simulink model "DAL_Sat_HW_v5"  (R2021b)
settings: Solver=FixedStepAuto  StartTime=0.0  StopTime=Inf  RelTol=1e-3  EnableMultiTasking=on
undefined symbols (not defined in the file): magnitude
libraries: arduinolib x11
settings Model: ExtModeTrigDuration=2  Creator=diego  LastModifiedBy=diego
settings OptimizationCC: EnhancedBackFolding=on  PassReuseOutputArgsAs=Individual arguments  ZeroExternalMemoryAtStartup=off  ZeroInternalMemoryAtStartup=off  MaxStackSize=64  OptimizeBlockOrder=speed  DifferentSizesBufferReuse=on  EfficientTunableParamExpr=on
settings DebuggingCC: ParameterTunabilityLossMsg=error
settings HardwareCC: ProdBitPerInt=16  ProdBitPerPointer=16  ProdBitPerSizeT=16  ProdBitPerPtrDiffT=16  ProdLargestAtomicFloat=None  ProdWordSize=8  ProdHWDeviceType=Atmel->AVR
settings SFSimCC: MATLABDynamicMemAlloc=off
settings RTWCC: Description=Embedded Coder  SystemTargetFile=ert.tlc  HardwareBoard=Arduino Uno  TemplateMakefile=ert_default_tmf  Toolchain=Arduino AVR  BuildConfiguration=Faster Runs
settings CodeAppCC: ForceParamTrailComments=on  IgnoreCustomStorageClasses=off  OperatorAnnotations=on  SimulinkDataObjDesc=on  SFDataObjDesc=on  InsertBlockDesc=on
settings ERTTargetCC: SupportContinuousTime=on  SupportVariableSizeSignals=on  ExtModeTransport=3  ExtModeStaticAlloc=on  ExtModeStaticAllocSize=250  ExtModeMexFile=ext_xcp  ExtModeIntrfLevel=Level2 - Open

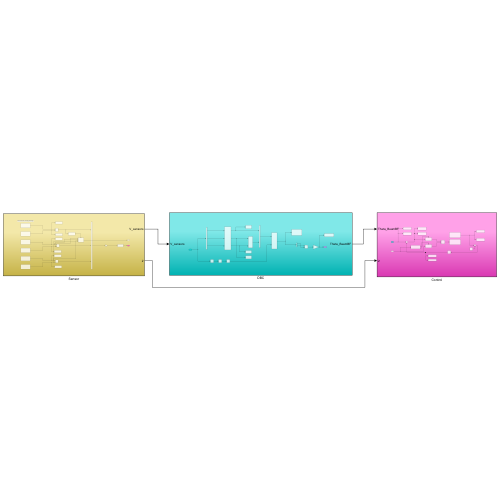
[thumbnail: Simulink's stored preview of the top-level diagram]
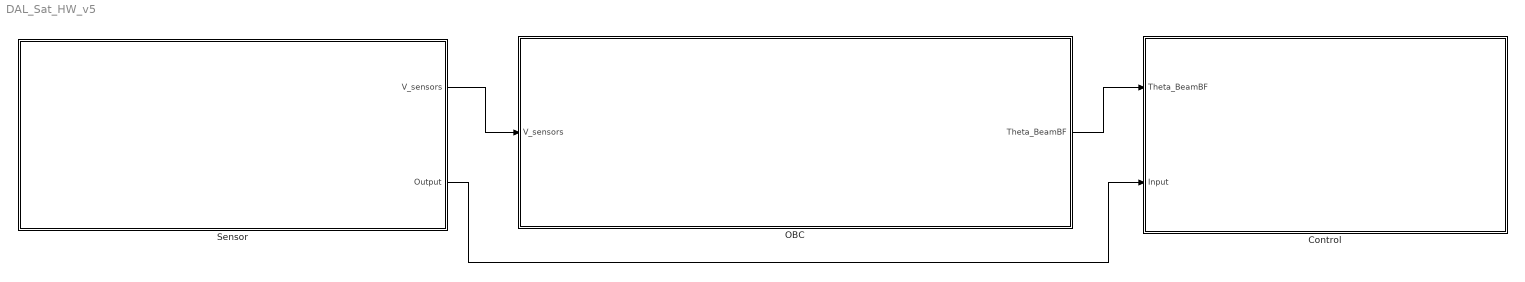
== system DAL_Sat_HW_v5 ==
  Control : Subsystem
  OBC : Subsystem
  Sensor : Subsystem
  wires:
  OBC/1(Theta_BeamBF) -> Control/1(Theta_BeamBF)
  Sensor/1(V_sensors) -> OBC/1(V_sensors)
  Sensor/2(Output) -> Control/2(Input)

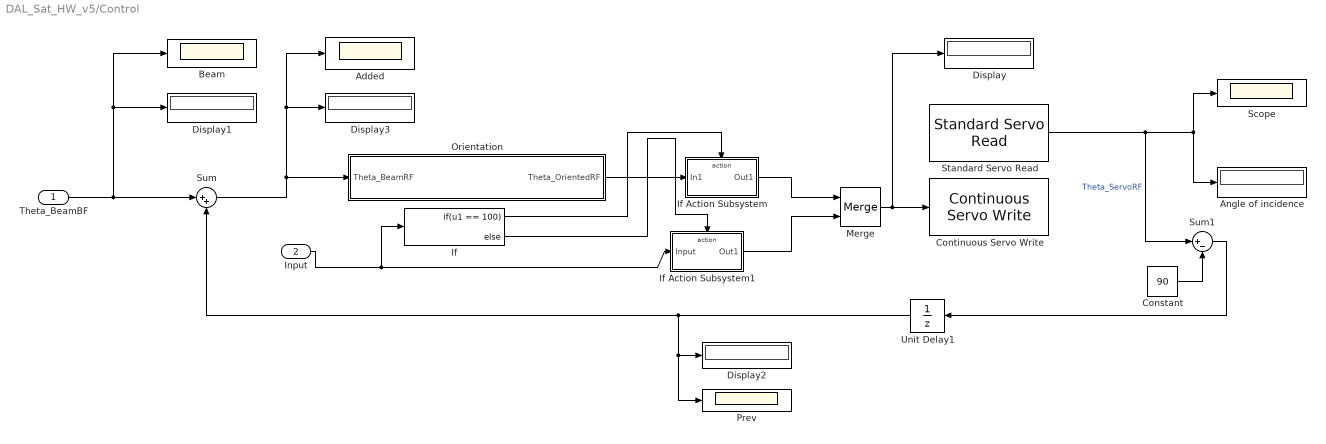
== system DAL_Sat_HW_v5/Control ==
  Theta_BeamBF : Inport
  Input : Inport  Port=2
  Added : Scope
  Angle of incidence : Display
  Beam : Scope
  Constant : Constant  Value=90
  Continuous Servo Write : arduinolib/Continuous Servo Write  pinNumber=9  ServoIndex=0  blockPlatform=ARDUINO
      settings: SourceProductBaseCode=ARDUINO
  Display{,1..3} (4 alike) : Display
  If : If  IfExpression=u1 == 100
  If Action Subsystem : Subsystem  TreatAsAtomicUnit=on
  If Action Subsystem1 : Subsystem  TreatAsAtomicUnit=on
  Merge : Merge
  Orientation : Subsystem
  Prev : Scope
  Scope : Scope
  Standard Servo Read : arduinolib/Standard Servo Read  pinNumber=9  SampleTime=0.1  ServoIndex=0  blockPlatform=ARDUINO
      settings: SourceProductBaseCode=ARDUINO
  Sum : Sum  Inputs=|++
  Sum1 : Sum  Inputs=|+-
  Unit Delay1 : UnitDelay  SampleTime=-1  HasFrameUpgradeWarning=on
  wires:
  Standard Servo Read/1 -> Scope/1, Angle of incidence/1, Sum1/1  "Theta_ServoRF"
  Unit Delay1/1 -> Prev/1, Display2/1, Sum/2
  Theta_BeamBF/1 -> Beam/1, Display1/1, Sum/1
  Sum1/1 -> Unit Delay1/1
  Constant/1 -> Sum1/2
  Sum/1 -> Display3/1, Added/1, Orientation/1(Theta_BeamRF)
  Merge/1 -> Display/1, Continuous Servo Write/1
  Input/1 -> If/1, If Action Subsystem1/1(Input)
  If/1 -> If Action Subsystem/Action
  If/2 -> If Action Subsystem1/Action
  If Action Subsystem/1(Out1) -> Merge/1
  If Action Subsystem1/1(Out1) -> Merge/2
  Orientation/1(Theta_OrientedRF) -> If Action Subsystem/1(In1)

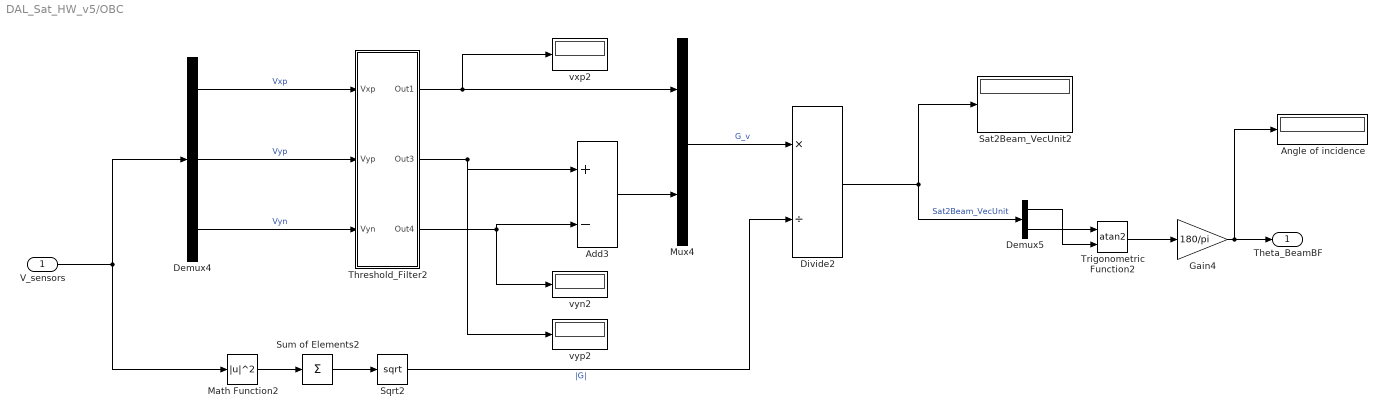
== system DAL_Sat_HW_v5/OBC ==
  V_sensors : Inport
  Add3 : Sum  Inputs=+|-
  Angle of incidence : Display
  Demux4 : Demux  Outputs=3
  Demux5 : Demux  Outputs=2
  Divide2 : Product  Inputs=*/
  Gain4 : Gain  Gain=180/pi
  Math Function2 : Math  Operator=magnitude^2  OutputSignalType=real  SaturateOnIntegerOverflow=on
  Mux4 : Mux  Inputs=2
  Sat2Beam_VecUnit2 : Display
  Sqrt2 : Sqrt  SaturateOnIntegerOverflow=on
  Sum of Elements2 : Sum  Inputs=+
  Threshold_Filter2 : Subsystem
  Trigonometric Function2 : Trigonometry  Operator=atan2
  vxp2 : Display
  vyn2 : Display
  vyp2 : Display
  Theta_BeamBF : Outport
  wires:
  V_sensors/1 -> Demux4/1, Math Function2/1
  Demux4/2 -> Threshold_Filter2/2(Vyp)  "Vyp"
  Trigonometric Function2/1 -> Gain4/1
  Threshold_Filter2/1(Out1) -> vxp2/1, Mux4/1
  Divide2/1 -> Sat2Beam_VecUnit2/1, Demux5/1  "Sat2Beam_VecUnit"
  Demux4/3 -> Threshold_Filter2/3(Vyn)  "Vyn"
  Sqrt2/1 -> Divide2/2  "|G|"
  Demux5/1 -> Trigonometric Function2/2
  Demux4/1 -> Threshold_Filter2/1(Vxp)  "Vxp"
  Threshold_Filter2/3(Out4) -> vyn2/1, Add3/2
  Add3/1 -> Mux4/2
  Threshold_Filter2/2(Out3) -> vyp2/1, Add3/1
  Mux4/1 -> Divide2/1  "G_v"
  Demux5/2 -> Trigonometric Function2/1
  Sum of Elements2/1 -> Sqrt2/1
  Math Function2/1 -> Sum of Elements2/1
  Gain4/1 -> Angle of incidence/1, Theta_BeamBF/1

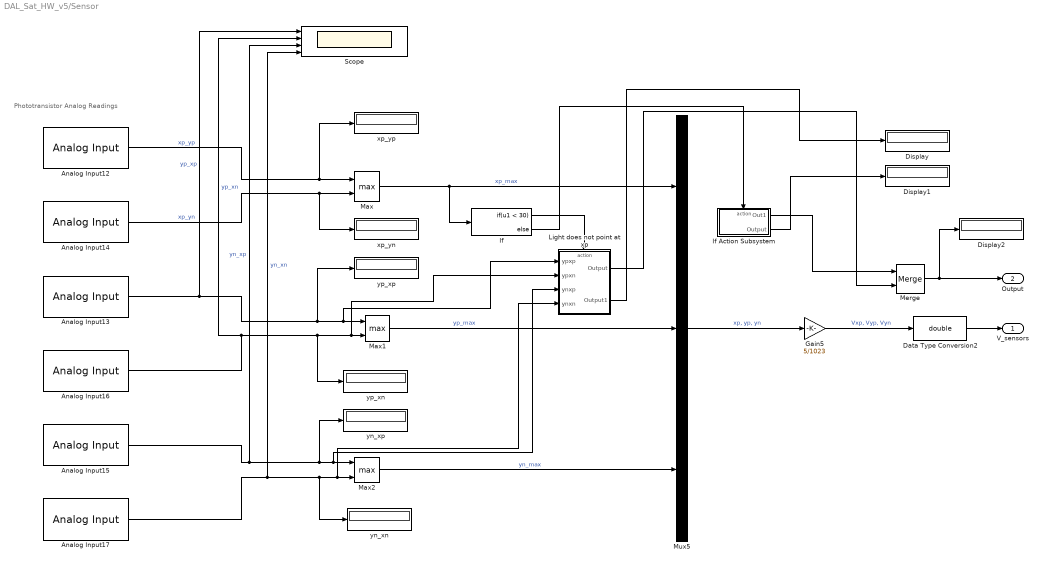
== system DAL_Sat_HW_v5/Sensor ==
  note: Phototransistor Analog Readings
  Analog Input12 : arduinolib/Analog Input  pinNumber=2  ReadResultsOnly=off  ConversionTriggerSource=Software  ExternalTriggerType=uint32( 0 )  OutputDataType=uint16  EnableConversionCompleteNotify=off  EnableOuputStatus=off  SampleTime=-1  blockPlatform=arduino
  Analog Input13 : arduinolib/Analog Input  pinNumber=1  ReadResultsOnly=off  ConversionTriggerSource=Software  ExternalTriggerType=uint32( 0 )  OutputDataType=uint16  EnableConversionCompleteNotify=off  EnableOuputStatus=off  SampleTime=-1  blockPlatform=arduino
  Analog Input14 : arduinolib/Analog Input  pinNumber=3  ReadResultsOnly=off  ConversionTriggerSource=Software  ExternalTriggerType=uint32( 0 )  OutputDataType=uint16  EnableConversionCompleteNotify=off  EnableOuputStatus=off  SampleTime=-1  blockPlatform=arduino
  Analog Input15 : arduinolib/Analog Input  pinNumber=4  ReadResultsOnly=off  ConversionTriggerSource=Software  ExternalTriggerType=uint32( 0 )  OutputDataType=uint16  EnableConversionCompleteNotify=off  EnableOuputStatus=off  SampleTime=-1  blockPlatform=arduino
  Analog Input16 : arduinolib/Analog Input  pinNumber=0  ReadResultsOnly=off  ConversionTriggerSource=Software  ExternalTriggerType=uint32( 0 )  OutputDataType=uint16  EnableConversionCompleteNotify=off  EnableOuputStatus=off  SampleTime=-1  blockPlatform=arduino
  Analog Input17 : arduinolib/Analog Input  pinNumber=5  ReadResultsOnly=off  ConversionTriggerSource=Software  ExternalTriggerType=uint32( 0 )  OutputDataType=uint16  EnableConversionCompleteNotify=off  EnableOuputStatus=off  SampleTime=-1  blockPlatform=arduino
  Data Type Conversion2 : DataTypeConversion  OutDataTypeStr=double
  Display : Display
  Display1 : Display
  Display2 : Display
  Gain5 : Gain  Gain=5/1023
  If : If  IfExpression=u1 < 30
  If Action Subsystem : Subsystem  TreatAsAtomicUnit=on
  Light does not point at xp : Subsystem  TreatAsAtomicUnit=on
  Max : MinMax  Function=max  Inputs=2
  Max1 : MinMax  Function=max  Inputs=2
  Max2 : MinMax  Function=max  Inputs=2
  Merge : Merge
  Mux5 : Mux  Inputs=3
  Scope : Scope  NumInputPorts=4
  xp_yn : Display
  xp_yp : Display
  yn_xn : Display
  yn_xp : Display
  yp_xn : Display
  yp_xp : Display
  V_sensors : Outport
  Output : Outport  Port=2
  wires:
  Analog Input12/1 -> Max/1, xp_yp/1  "xp_yp"
  Analog Input14/1 -> Max/2, xp_yn/1  "xp_yn"
  Analog Input13/1 -> Light does not point at xp/1(ypxp), Max1/1, yp_xp/1, Scope/1  "yp_xp"
  Max2/1 -> Mux5/3  "yn_max"
  Max/1 -> If/1, Mux5/1  "xp_max"
  Analog Input15/1 -> Light does not point at xp/3(ynxp), Max2/1, yn_xp/1, Scope/3  "yn_xp"
  Analog Input16/1 -> Light does not point at xp/2(ypxn), Max1/2, yp_xn/1, Scope/2  "yp_xn"
  Analog Input17/1 -> Light does not point at xp/4(ynxn), Max2/2, yn_xn/1, Scope/4  "yn_xn"
  Max1/1 -> Mux5/2  "yp_max"
  Mux5/1 -> Gain5/1  "xp, yp, yn"
  Gain5/1 -> Data Type Conversion2/1  "Vxp, Vyp, Vyn"
  Data Type Conversion2/1 -> V_sensors/1
  If/1 -> Light does not point at xp/Action
  Merge/1 -> Display2/1, Output/1
  If Action Subsystem/1(Out1) -> Merge/1
  Light does not point at xp/1(Output) -> Merge/2
  If/2 -> If Action Subsystem/Action
  Light does not point at xp/2(Output1) -> Display/1
  If Action Subsystem/2(Output) -> Display1/1

== system DAL_Sat_HW_v5/Control/If Action Subsystem ==
  In1 : Inport
  Action Port : ActionPort  ActionPortLabel=if(u1 == 100)
  Out1 : Outport
  wires:
  In1/1 -> Out1/1

== system DAL_Sat_HW_v5/Control/If Action Subsystem1 ==
  Input : Inport
  Action Port : ActionPort  ActionPortLabel=else
  Out1 : Outport
  wires:
  Input/1 -> Out1/1

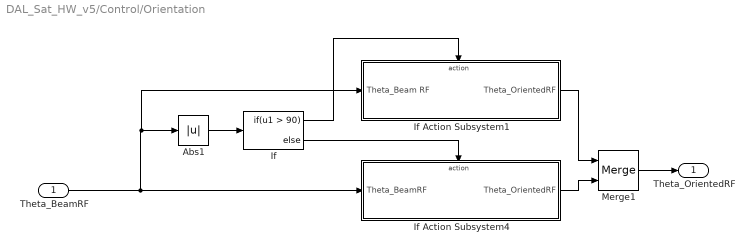
== system DAL_Sat_HW_v5/Control/Orientation ==
  Theta_BeamRF : Inport
  Abs1 : Abs
  If : If  IfExpression=u1 > 90
  If Action Subsystem1 : Subsystem  TreatAsAtomicUnit=on
  If Action Subsystem4 : Subsystem  TreatAsAtomicUnit=on
  Merge1 : Merge
  Theta_OrientedRF : Outport
  wires:
  If Action Subsystem1/1(Theta_OrientedRF) -> Merge1/1
  Merge1/1 -> Theta_OrientedRF/1
  If/2 -> If Action Subsystem4/Action
  If/1 -> If Action Subsystem1/Action
  Abs1/1 -> If/1
  Theta_BeamRF/1 -> If Action Subsystem1/1(Theta_Beam	RF), Abs1/1, If Action Subsystem4/1(Theta_BeamRF)
  If Action Subsystem4/1(Theta_OrientedRF) -> Merge1/2

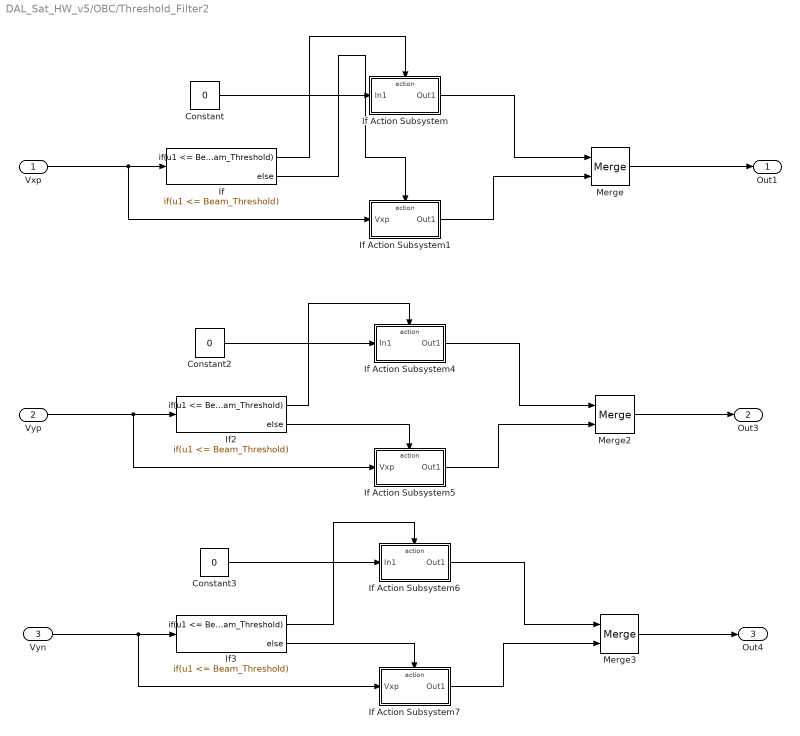
== system DAL_Sat_HW_v5/OBC/Threshold_Filter2 ==
  Vxp : Inport
  Vyp : Inport  Port=2
  Vyn : Inport  Port=3
  Constant : Constant  Value=0
  Constant2 : Constant  Value=0
  Constant3 : Constant  Value=0
  If : If  IfExpression=u1 <= Beam_Threshold
  If Action Subsystem : Subsystem  TreatAsAtomicUnit=on
  If Action Subsystem1 : Subsystem  TreatAsAtomicUnit=on
  If Action Subsystem4 : Subsystem  TreatAsAtomicUnit=on
  If Action Subsystem5 : Subsystem  TreatAsAtomicUnit=on
  If Action Subsystem6 : Subsystem  TreatAsAtomicUnit=on
  If Action Subsystem7 : Subsystem  TreatAsAtomicUnit=on
  If2 : If  IfExpression=u1 <= Beam_Threshold
  If3 : If  IfExpression=u1 <= Beam_Threshold
  Merge : Merge
  Merge2 : Merge
  Merge3 : Merge
  Out1 : Outport
  Out3 : Outport  Port=2
  Out4 : Outport  Port=3
  wires:
  Vxp/1 -> If Action Subsystem1/1(Vxp), If/1
  If/1 -> If Action Subsystem/Action
  If Action Subsystem/1(Out1) -> Merge/1
  If/2 -> If Action Subsystem1/Action
  If Action Subsystem1/1(Out1) -> Merge/2
  Merge/1 -> Out1/1
  Constant/1 -> If Action Subsystem/1(In1)
  Vyp/1 -> If2/1, If Action Subsystem5/1(Vxp)
  If2/2 -> If Action Subsystem5/Action
  If2/1 -> If Action Subsystem4/Action
  If Action Subsystem4/1(Out1) -> Merge2/1
  If Action Subsystem5/1(Out1) -> Merge2/2
  Constant2/1 -> If Action Subsystem4/1(In1)
  Merge2/1 -> Out3/1
  Vyn/1 -> If3/1, If Action Subsystem7/1(Vxp)
  Merge3/1 -> Out4/1
  If Action Subsystem7/1(Out1) -> Merge3/2
  If3/2 -> If Action Subsystem7/Action
  If Action Subsystem6/1(Out1) -> Merge3/1
  Constant3/1 -> If Action Subsystem6/1(In1)
  If3/1 -> If Action Subsystem6/Action

== system DAL_Sat_HW_v5/Sensor/If Action Subsystem ==
  Action Port : ActionPort  ActionPortLabel=else
  Constant : Constant  Value=100
  Out1 : Outport
  Output : Outport  Port=2
  wires:
  Constant/1 -> Output/1, Out1/1

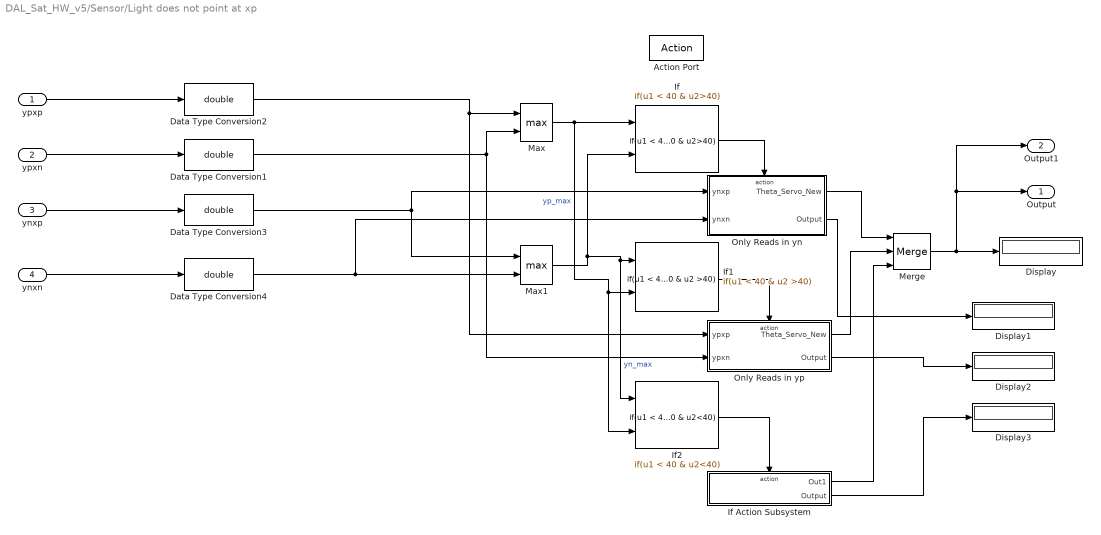
== system DAL_Sat_HW_v5/Sensor/Light does not point at xp ==
  ypxp : Inport
  ypxn : Inport  Port=2
  ynxp : Inport  Port=3
  ynxn : Inport  Port=4
  Action Port : ActionPort  ActionPortLabel=if(u1 < 30)
  Data Type Conversion{1..4} (4 alike) : DataTypeConversion  OutDataTypeStr=double
  Display{,1..3} (4 alike) : Display
  If : If  NumInputs=2  IfExpression=u1 < 40 & u2>40  ShowElse=off
  If Action Subsystem : Subsystem  TreatAsAtomicUnit=on
  If1 : If  NumInputs=2  IfExpression=u1 < 40 & u2 >40  ShowElse=off
  If2 : If  NumInputs=2  IfExpression=u1 < 40 & u2<40  ShowElse=off
  Max : MinMax  Function=max  Inputs=2
  Max1 : MinMax  Function=max  Inputs=2
  Merge : Merge  Inputs=3
  Only Reads in yn : Subsystem  TreatAsAtomicUnit=on
  Only Reads in yp : Subsystem  TreatAsAtomicUnit=on
  Output : Outport
  Output1 : Outport  Port=2
  wires:
  Max/1 -> If2/2, If1/2, If/1  "yp_max"
  Max1/1 -> If/2, If2/1, If1/1  "yn_max"
  Only Reads in yn/1(Theta_Servo_New) -> Merge/1
  Only Reads in yp/1(Theta_Servo_New) -> Merge/2
  Merge/1 -> Output1/1, Output/1, Display/1
  If/1 -> Only Reads in yn/Action
  If1/1 -> Only Reads in yp/Action
  If2/1 -> If Action Subsystem/Action
  If Action Subsystem/1(Out1) -> Merge/3
  Only Reads in yn/2(Output) -> Display1/1
  Only Reads in yp/2(Output) -> Display2/1
  If Action Subsystem/2(Output) -> Display3/1
  Data Type Conversion2/1 -> Only Reads in yp/1(ypxp), Max/1
  Data Type Conversion1/1 -> Only Reads in yp/2(ypxn), Max/2
  Data Type Conversion3/1 -> Max1/1, Only Reads in yn/1(ynxp)
  ypxn/1 -> Data Type Conversion1/1
  ypxp/1 -> Data Type Conversion2/1
  ynxn/1 -> Data Type Conversion4/1
  ynxp/1 -> Data Type Conversion3/1
  Data Type Conversion4/1 -> Only Reads in yn/2(ynxn), Max1/2

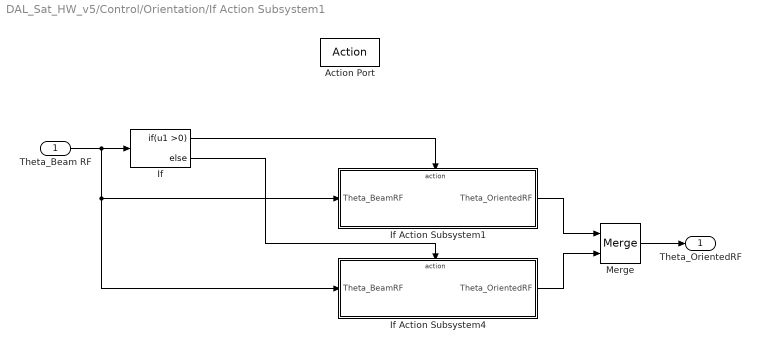
== system DAL_Sat_HW_v5/Control/Orientation/If Action Subsystem1 ==
  Theta_Beam	RF : Inport
  Action Port : ActionPort  ActionPortLabel=if(u1 > 90)
  If : If  IfExpression=u1 >0
  If Action Subsystem1 : Subsystem  TreatAsAtomicUnit=on
  If Action Subsystem4 : Subsystem  TreatAsAtomicUnit=on
  Merge : Merge
  Theta_OrientedRF : Outport
  wires:
  Theta_Beam	RF/1 -> If Action Subsystem4/1(Theta_BeamRF), If Action Subsystem1/1(Theta_BeamRF), If/1
  If/1 -> If Action Subsystem1/Action
  If/2 -> If Action Subsystem4/Action
  If Action Subsystem1/1(Theta_OrientedRF) -> Merge/1
  If Action Subsystem4/1(Theta_OrientedRF) -> Merge/2
  Merge/1 -> Theta_OrientedRF/1

== system DAL_Sat_HW_v5/Control/Orientation/If Action Subsystem4 ==
  Theta_BeamRF : Inport
  Action Port : ActionPort  ActionPortLabel=else
  Theta_OrientedRF : Outport
  wires:
  Theta_BeamRF/1 -> Theta_OrientedRF/1

== system DAL_Sat_HW_v5/OBC/Threshold_Filter2/If Action Subsystem ==
  In1 : Inport
  Action Port : ActionPort  ActionPortLabel=if(u1 <= Beam_Threshold)
  Out1 : Outport
  wires:
  In1/1 -> Out1/1

== system DAL_Sat_HW_v5/OBC/Threshold_Filter2/If Action Subsystem1 ==
  Vxp : Inport
  Action Port : ActionPort  ActionPortLabel=else
  Out1 : Outport
  wires:
  Vxp/1 -> Out1/1

== system DAL_Sat_HW_v5/OBC/Threshold_Filter2/If Action Subsystem4 ==
  In1 : Inport
  Action Port : ActionPort  ActionPortLabel=if(u1 <= Beam_Threshold)
  Out1 : Outport
  wires:
  In1/1 -> Out1/1

== system DAL_Sat_HW_v5/OBC/Threshold_Filter2/If Action Subsystem5 ==
  Vxp : Inport
  Action Port : ActionPort  ActionPortLabel=else
  Out1 : Outport
  wires:
  Vxp/1 -> Out1/1

== system DAL_Sat_HW_v5/OBC/Threshold_Filter2/If Action Subsystem6 ==
  In1 : Inport
  Action Port : ActionPort  ActionPortLabel=if(u1 <= Beam_Threshold)
  Out1 : Outport
  wires:
  In1/1 -> Out1/1

== system DAL_Sat_HW_v5/OBC/Threshold_Filter2/If Action Subsystem7 ==
  Vxp : Inport
  Action Port : ActionPort  ActionPortLabel=else
  Out1 : Outport
  wires:
  Vxp/1 -> Out1/1

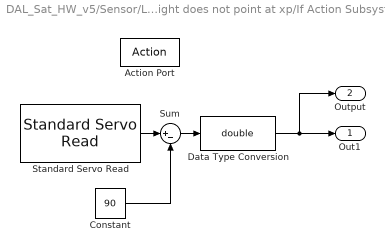
== system DAL_Sat_HW_v5/Sensor/Light does not point at xp/If Action Subsystem ==
  Action Port : ActionPort  ActionPortLabel=if(u1 < 40 & u2<40)
  Constant : Constant  Value=90
  Data Type Conversion : DataTypeConversion  OutDataTypeStr=double
  Standard Servo Read : arduinolib/Standard Servo Read  pinNumber=2  SampleTime=0.1  ServoIndex=1  blockPlatform=ARDUINO
      settings: SourceProductBaseCode=ARDUINO
  Sum : Sum  Inputs=|+-
  Out1 : Outport
  Output : Outport  Port=2
  wires:
  Data Type Conversion/1 -> Output/1, Out1/1
  Standard Servo Read/1 -> Sum/1
  Sum/1 -> Data Type Conversion/1
  Constant/1 -> Sum/2

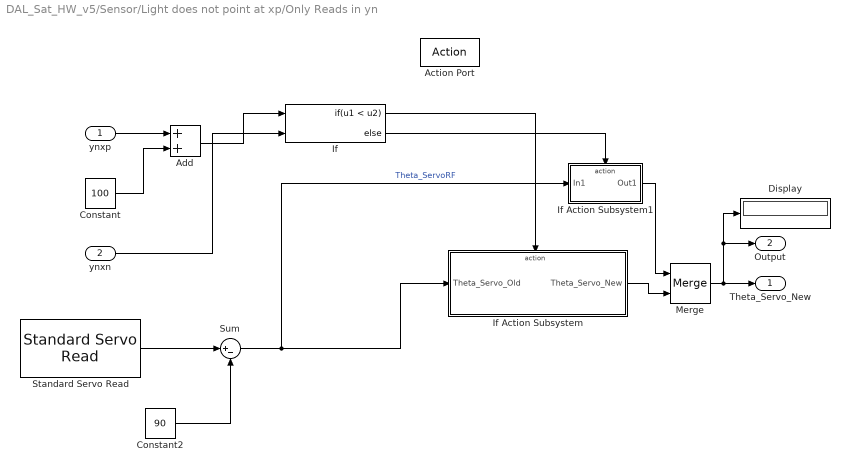
== system DAL_Sat_HW_v5/Sensor/Light does not point at xp/Only Reads in yn ==
  ynxp : Inport
  ynxn : Inport  Port=2
  Action Port : ActionPort  ActionPortLabel=if(u1 < 40 & u2>40)
  Add : Sum
  Constant : Constant  Value=100
  Constant2 : Constant  Value=90
  Display : Display
  If : If  NumInputs=2  IfExpression=u1 < u2
  If Action Subsystem : Subsystem  TreatAsAtomicUnit=on
  If Action Subsystem1 : Subsystem  TreatAsAtomicUnit=on
  Merge : Merge
  Standard Servo Read : arduinolib/Standard Servo Read  pinNumber=9  SampleTime=0.1  ServoIndex=0  blockPlatform=ARDUINO
      settings: SourceProductBaseCode=ARDUINO
  Sum : Sum  Inputs=|+-
  Theta_Servo_New : Outport
  Output : Outport  Port=2
  wires:
  ynxp/1 -> Add/1
  Constant/1 -> Add/2
  Add/1 -> If/1
  ynxn/1 -> If/2
  If/1 -> If Action Subsystem/Action
  If/2 -> If Action Subsystem1/Action
  If Action Subsystem1/1(Out1) -> Merge/1
  If Action Subsystem/1(Theta_Servo_New) -> Merge/2
  Merge/1 -> Display/1, Output/1, Theta_Servo_New/1
  Standard Servo Read/1 -> Sum/1
  Sum/1 -> If Action Subsystem1/1(In1), If Action Subsystem/1(Theta_Servo_Old)  "Theta_ServoRF"
  Constant2/1 -> Sum/2

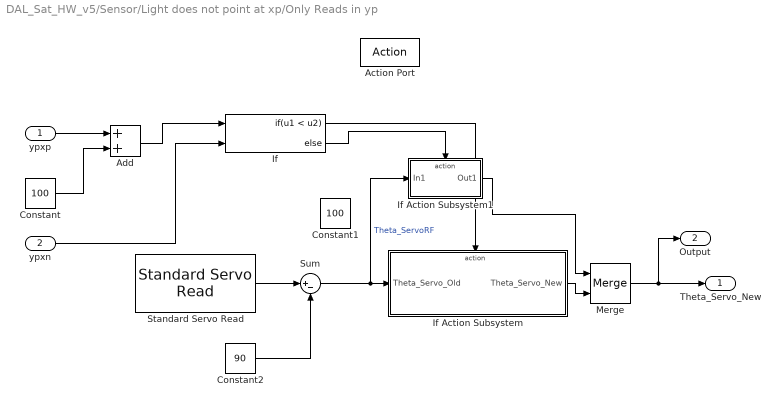
== system DAL_Sat_HW_v5/Sensor/Light does not point at xp/Only Reads in yp ==
  ypxp : Inport
  ypxn : Inport  Port=2
  Action Port : ActionPort  ActionPortLabel=if(u1 < 40 & u2 >40)
  Add : Sum
  Constant : Constant  Value=100
  Constant1 : Constant  Value=100
  Constant2 : Constant  Value=90
  If : If  NumInputs=2  IfExpression=u1 < u2
  If Action Subsystem : Subsystem  TreatAsAtomicUnit=on
  If Action Subsystem1 : Subsystem  TreatAsAtomicUnit=on
  Merge : Merge
  Standard Servo Read : arduinolib/Standard Servo Read  pinNumber=9  SampleTime=0.1  ServoIndex=0  blockPlatform=ARDUINO
      settings: SourceProductBaseCode=ARDUINO
  Sum : Sum  Inputs=|+-
  Theta_Servo_New : Outport
  Output : Outport  Port=2
  wires:
  ypxp/1 -> Add/1
  Constant/1 -> Add/2
  Add/1 -> If/1
  ypxn/1 -> If/2
  If/1 -> If Action Subsystem/Action
  If/2 -> If Action Subsystem1/Action
  Merge/1 -> Output/1, Theta_Servo_New/1
  If Action Subsystem1/1(Out1) -> Merge/1
  If Action Subsystem/1(Theta_Servo_New) -> Merge/2
  Sum/1 -> If Action Subsystem1/1(In1), If Action Subsystem/1(Theta_Servo_Old)  "Theta_ServoRF"
  Standard Servo Read/1 -> Sum/1
  Constant2/1 -> Sum/2

== system DAL_Sat_HW_v5/Control/Orientation/If Action Subsystem1/If Action Subsystem1 ==
  Theta_BeamRF : Inport
  Action Port : ActionPort  ActionPortLabel=if(u1 >0)
  Constant : Constant  Value=180
  Subtract : Sum
  Theta_OrientedRF : Outport
  wires:
  Subtract/1 -> Theta_OrientedRF/1
  Theta_BeamRF/1 -> Subtract/1
  Constant/1 -> Subtract/2

== system DAL_Sat_HW_v5/Control/Orientation/If Action Subsystem1/If Action Subsystem4 ==
  Theta_BeamRF : Inport
  Action Port : ActionPort  ActionPortLabel=else
  Constant : Constant  Value=180
  Subtract : Sum  Inputs=+-
  Theta_OrientedRF : Outport
  wires:
  Theta_BeamRF/1 -> Subtract/1
  Constant/1 -> Subtract/2
  Subtract/1 -> Theta_OrientedRF/1

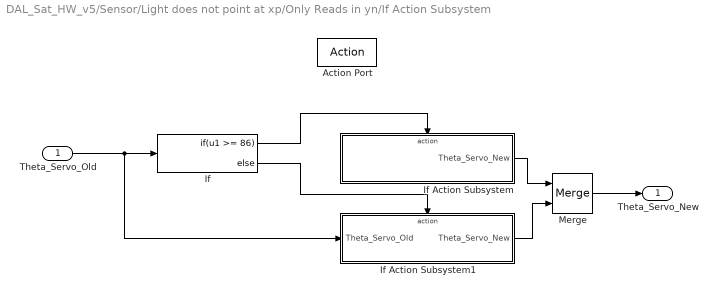
== system DAL_Sat_HW_v5/Sensor/Light does not point at xp/Only Reads in yn/If Action Subsystem ==
  Theta_Servo_Old : Inport
  Action Port : ActionPort  ActionPortLabel=if(u1 < u2)
  If : If  IfExpression=u1 >= 86
  If Action Subsystem : Subsystem  TreatAsAtomicUnit=on
  If Action Subsystem1 : Subsystem  TreatAsAtomicUnit=on
  Merge : Merge
  Theta_Servo_New : Outport
  wires:
  Theta_Servo_Old/1 -> If Action Subsystem1/1(Theta_Servo_Old), If/1
  If/2 -> If Action Subsystem1/Action
  If Action Subsystem/1(Theta_Servo_New) -> Merge/1
  If Action Subsystem1/1(Theta_Servo_New) -> Merge/2
  Merge/1 -> Theta_Servo_New/1
  If/1 -> If Action Subsystem/Action

== system DAL_Sat_HW_v5/Sensor/Light does not point at xp/Only Reads in yn/If Action Subsystem1 ==
  In1 : Inport
  Action Port : ActionPort  ActionPortLabel=else
  Out1 : Outport
  wires:
  In1/1 -> Out1/1

== system DAL_Sat_HW_v5/Sensor/Light does not point at xp/Only Reads in yp/If Action Subsystem ==
  Theta_Servo_Old : Inport
  Action Port : ActionPort  ActionPortLabel=if(u1 < u2)
  If : If  IfExpression=u1 <= -86
  If Action Subsystem : Subsystem  TreatAsAtomicUnit=on
  If Action Subsystem1 : Subsystem  TreatAsAtomicUnit=on
  Merge : Merge
  Theta_Servo_New : Outport
  wires:
  Theta_Servo_Old/1 -> If Action Subsystem1/1(Theta_Servo_Old), If/1
  If Action Subsystem/1(Theta_Servo_New) -> Merge/1
  If Action Subsystem1/1(Theta_Servo_New) -> Merge/2
  Merge/1 -> Theta_Servo_New/1
  If/2 -> If Action Subsystem1/Action
  If/1 -> If Action Subsystem/Action

== system DAL_Sat_HW_v5/Sensor/Light does not point at xp/Only Reads in yp/If Action Subsystem1 ==
  In1 : Inport
  Action Port : ActionPort  ActionPortLabel=else
  Out1 : Outport
  wires:
  In1/1 -> Out1/1

== system DAL_Sat_HW_v5/Sensor/Light does not point at xp/Only Reads in yn/If Action Subsystem/If Action Subsystem ==
  Action Port : ActionPort  ActionPortLabel=if(u1 >= 86)
  Constant : Constant  Value=-90
  Theta_Servo_New : Outport
  wires:
  Constant/1 -> Theta_Servo_New/1

== system DAL_Sat_HW_v5/Sensor/Light does not point at xp/Only Reads in yn/If Action Subsystem/If Action Subsystem1 ==
  Theta_Servo_Old : Inport
  Action Port : ActionPort  ActionPortLabel=else
  Add : Sum
  Constant : Constant  Value=5
  Theta_Servo_New : Outport
  wires:
  Theta_Servo_Old/1 -> Add/1
  Add/1 -> Theta_Servo_New/1
  Constant/1 -> Add/2

== system DAL_Sat_HW_v5/Sensor/Light does not point at xp/Only Reads in yp/If Action Subsystem/If Action Subsystem ==
  Action Port : ActionPort  ActionPortLabel=if(u1 <= -86)
  Constant : Constant  Value=90
  Theta_Servo_New : Outport
  wires:
  Constant/1 -> Theta_Servo_New/1

== system DAL_Sat_HW_v5/Sensor/Light does not point at xp/Only Reads in yp/If Action Subsystem/If Action Subsystem1 ==
  Theta_Servo_Old : Inport
  Action Port : ActionPort  ActionPortLabel=else
  Add : Sum  Inputs=+-
  Constant : Constant  Value=5
  Theta_Servo_New : Outport
  wires:
  Theta_Servo_Old/1 -> Add/1
  Add/1 -> Theta_Servo_New/1
  Constant/1 -> Add/2
